simulink model "Tx"  (R2018b)
settings: Solver=VariableStepAuto  StartTime=0.0  StopTime=10.0  RelTol=1e-3
libraries: pePwmGenerator x1, dspnetwork x1
settings Model: xpc_rtwmakecfg_data=_xpcetherlib__xpcether8255xlib__xpcetherGbElib__xpciplib__xpcnblib_  EnablePacing=on  Creator=79301  LastModifiedBy=79301

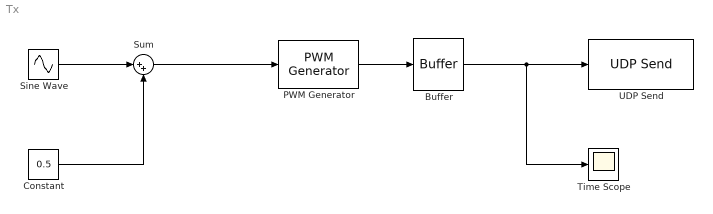
== system Tx ==
  Buffer : Buffer  N=4096  OutputFrames=off
  Constant : Constant  Value=0.5  SampleTime=0.0001
  PWM Generator : pePwmGenerator/PWM Generator  CarrCount=Up  Tper=0.001  Ts=0.0001
  Sine Wave : Sin  Amplitude=0.5  Frequency=100*pi  SampleTime=0.0001
  Sum : Sum  Inputs=|++
  Time Scope : Scope
  UDP Send : dspnetwork/UDP Send  remoteURL='255.255.255.255'  remotePort=25000  localURL='0.0.0.0'  localPortSource=Automatically determine  localPort=-1  sampletime=-1  blockPlatform=[]  separateLengthPort=0
      settings: SourceProductName=DSP System Toolbox  SourceProductBaseCode=DS
  wires:
  PWM Generator/1 -> Buffer/1
  Constant/1 -> Sum/2
  Sine Wave/1 -> Sum/1
  Sum/1 -> PWM Generator/1
  Buffer/1 -> Time Scope/1, UDP Send/1
